simulink model "drone_z_simulation"  (R2020a)
settings: Solver=FixedStepAuto  StartTime=0.0  StopTime=10.0  FixedStep=0.005  RelTol=1e-3
undefined symbols (not defined in the file or in its folder): DiscIntNeverNeededParam
settings Model: Creator=Ken  LastModifiedBy=denjo

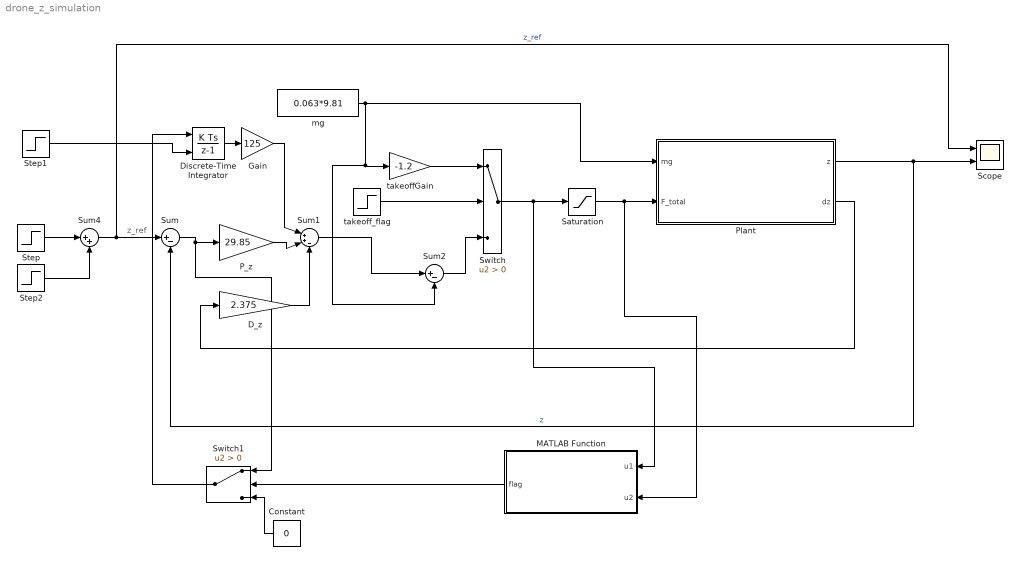
== system drone_z_simulation ==
  note: z_ref
  Constant : Constant  Value=0
  D_z : Gain  Gain=2.375
  Discrete-Time Integrator : DiscreteIntegrator  ExternalReset=rising  SampleTime=-1  ICPrevOutput=DiscIntNeverNeededParam  ICPrevScaledInput=DiscIntNeverNeededParam
  Gain : Gain  Gain=125
  MATLAB Function : MATLAB Function  TreatAsAtomicUnit=on
  P_z : Gain  Gain=29.85
  Plant : Subsystem
  Saturation : Saturate  UpperLimit=-0.026132  LowerLimit=-1.2020
  Scope : Scope  NumInputPorts=2
  Step : Step  After=-1.5  SampleTime=0
  Step1 : Step  SampleTime=0
  Step2 : Step  Time=5  After=-0.5  SampleTime=0
  Sum : Sum  Inputs=|+-
  Sum1 : Sum  Inputs=|++-
  Sum2 : Sum  Inputs=|+-
  Sum4 : Sum  Inputs=|++
  Switch : Switch  Criteria=u2 > Threshold
  Switch1 : Switch  Criteria=u2 > Threshold
  mg : Constant  Value=0.063*9.81
  takeoffGain : Gain  Gain=-1.2
  takeoff_flag : Step  Before=1  After=0  SampleTime=0
  wires:
  Sum4/1 -> Sum/1, Scope/1  "z_ref"
  Sum/1 -> Switch1/1, P_z/1
  P_z/1 -> Sum1/2
  D_z/1 -> Sum1/3
  mg/1 -> Plant/1(mg), Sum2/2, takeoffGain/1
  takeoffGain/1 -> Switch/1
  takeoff_flag/1 -> Switch/2
  Switch/1 -> Saturation/1, MATLAB Function/1(u1)
  Step/1 -> Sum4/1
  Step2/1 -> Sum4/2
  Plant/1(z) -> Scope/2, Sum/2  "z"
  Saturation/1 -> MATLAB Function/2(u2), Plant/2(F_total)
  Plant/2(dz) -> D_z/1
  Sum2/1 -> Switch/3
  Sum1/1 -> Sum2/1
  MATLAB Function/1(flag) -> Switch1/2
  Switch1/1 -> Discrete-Time Integrator/1
  Step1/1 -> Discrete-Time Integrator/2
  Discrete-Time Integrator/1 -> Gain/1
  Gain/1 -> Sum1/1
  Constant/1 -> Switch1/3

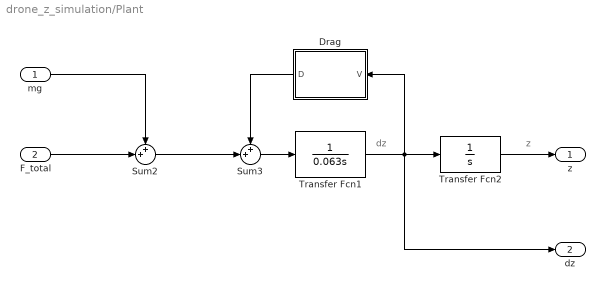
== system drone_z_simulation/Plant ==
  note: dz
  note: z
  mg : Inport
  F_total : Inport  Port=2
  Drag : MATLAB Function  TreatAsAtomicUnit=on
  Sum2 : Sum  Inputs=++|
  Sum3 : Sum  Inputs=++|
  Transfer Fcn1 : TransferFcn  Denominator=[0.063 0]
  Transfer Fcn2 : TransferFcn  Denominator=[1 0]
  z : Outport
  dz : Outport  Port=2
  wires:
  Transfer Fcn1/1 -> Drag/1(V), Transfer Fcn2/1, dz/1
  Drag/1(D) -> Sum3/1
  Sum2/1 -> Sum3/2
  mg/1 -> Sum2/1
  Sum3/1 -> Transfer Fcn1/1
  F_total/1 -> Sum2/2
  Transfer Fcn2/1 -> z/1

== matlab function drone_z_simulation/Plant/Drag ==
  data: V input; D output
function D = fcn(V)

rho = 1.1840;
S = 0.01;
C_d = 1.2;

q = 1/2*rho*V^2;

D = -1*sign(V)*C_d*q*S;

== matlab function drone_z_simulation/MATLAB Function ==
  data: u1 input; flag output; u2 input
function flag = fcn(u1,u2)
flag=-1
if u1==u2
    flag=1
end
